simulink model "sampleModel2432"  (R2017a)
settings: Solver=VariableStepAuto  StartTime=0.0  StopTime=10.0  RelTol=1e-3
undefined symbols (not defined in the file or in its folder): DiscIntNeverNeededParam, sigbuilder_block
libraries: simulink x354
(part 1 of 6)
settings Model: Creator=cyfuzz  LastModifiedBy=cyfuzz

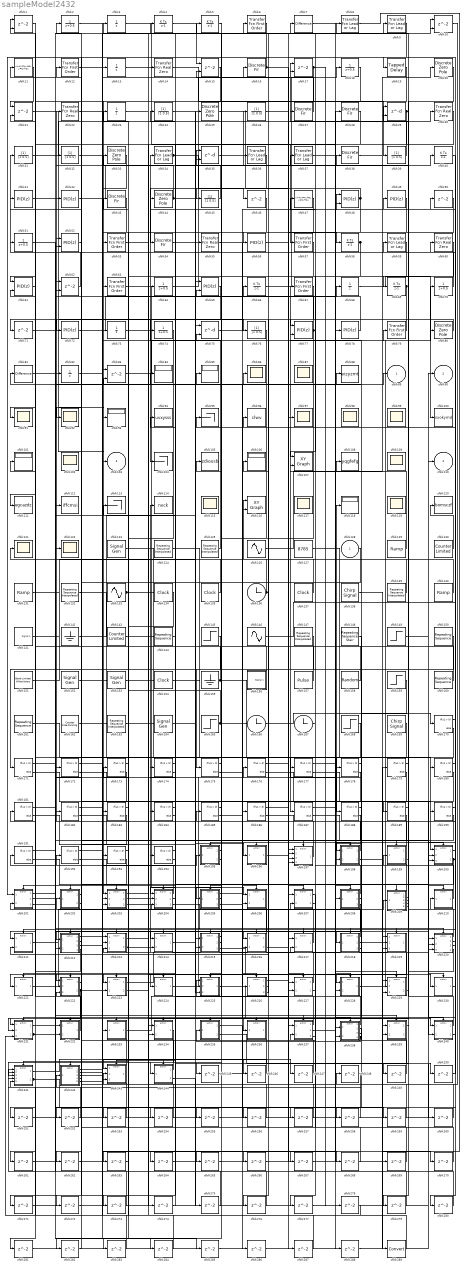
== system sampleModel2432 ==
  cfblk128 : Inport
  cfblk{1,10,15,17,21,62,83} (7 alike) : Delay  ShowEnablePort=on  SampleTime=1
      settings: InputPortMap=u0,e6
  cfblk100 : ToWorkspace  VariableName=sxokymd  SaveFormat=Timeseries  SampleTime=-1
  cfblk{84..85,93,101,106,118} (6 alike) : Display
  cfblk{86..87,91..92,97..99,102,109,115,117,119,121..122} (14 alike) : Scope
      cfblk102 settings: Floating=on
      cfblk109 settings: Floating=on
      cfblk115 settings: Floating=on
      cfblk117 settings: Floating=on
      cfblk119 settings: Floating=on
      cfblk87 settings: Floating=on
      cfblk98 settings: Floating=on
      cfblk99 settings: Floating=on
  cfblk104 : Terminator
  cfblk105 : ToWorkspace  VariableName=zdioxsb  SaveFormat=Timeseries  SampleTime=-1
  cfblk107 : simulink/Sinks/XY Graph  xmin=-1  xmax=1  ymin=-1  ymax=1  st=-1
  cfblk108 : ToWorkspace  VariableName=yqgfefg  SaveFormat=Timeseries  SampleTime=-1
  cfblk11 : DiscreteStateSpace
  cfblk111 : ToWorkspace  VariableName=egcazdz  SaveFormat=Timeseries  SampleTime=-1
  cfblk112 : ToWorkspace  VariableName=iffcmsi  SaveFormat=Timeseries  SampleTime=-1
  cfblk113 : Terminator
  cfblk114 : ToFile  Filename=nxck  SaveFormat=Timeseries
  cfblk116 : simulink/Sinks/XY Graph  xmin=-1  xmax=1  ymin=-1  ymax=1  st=-1
  cfblk{6,12,53,57,63,67,79} (7 alike) : simulink/Discrete/Transfer Fcn First Order  PoleZ=0.95  ICPrevOutput=0.0  DoSatur=off
      settings: SourceProductName=Simulink
  cfblk120 : ToWorkspace  VariableName=bomsczf  SaveFormat=Timeseries  SampleTime=-1
  cfblk{123,152..153,164} (4 alike) : SignalGenerator  Units=rad/sec
  cfblk{124..125,132,139,147,163} (6 alike) : simulink/Sources/Repeating Sequence Interpolated  OutValues=[3 1 4 2 1].'  TimeValues=[0 0.1 0.5 0.6 1].'  LookUpMeth=Interpolation-Use End Values  tsamp=0.01  OutMin=[]  OutMax=[]  OutDataTypeStr=double  OutputDataTypeScalingMode=double  OutDataType=fixdt(0,8)  OutScaling=2^-10
  cfblk126 : Sin  SampleTime=0
  cfblk127 : Constant  Value=8785
  cfblk129 : simulink/Sources/Ramp  slope=1  start=0  X0=0
  cfblk{3,13,23,68,73,82} (6 alike) : UnitDelay
  cfblk130 : simulink/Sources/Counter Limited  uplimit=7  tsamp=-1
  cfblk131 : simulink/Sources/Ramp  slope=1  start=0  X0=0
  cfblk133 : Sin  SampleTime=0
  cfblk{134..135,137,154} (4 alike) : DigitalClock
  cfblk136 : Clock
  cfblk138 : simulink/Sources/Chirp Signal  f1=0.1  T=100  f2=1
  cfblk{14,22,30,55,60} (5 alike) : simulink/Discrete/Transfer Fcn Real Zero  ZeroZ=0.75  ICPrevInput=0.0  DoSatur=off
      settings: SourceProductName=Simulink  SourceProductBaseCode=SL
  cfblk140 : simulink/Sources/Ramp  slope=1  start=0  X0=0
  cfblk141 : Subsystem  Tag=STV Subsys  LoadFcn=sigbuilder_block('load');  StartFcn=sigbuilder_block('start');  StopFcn=sigbuilder_block('stop');  ClipboardFcn=sigbuilder_block('clipboard');  mask(Sigbuilder block){tuvar=[0:10]}
      mask help: Simulink:masks:SigbuilderBlock_MD
      mask init:
      | if ~strcmp(get_param(bdroot(gcbh),'SimulationStatus'),'stopped') tuvar = sigbuilder_block('maskInit'); end
      settings: CopyFcn=sigbuilder_block('copy');  DeleteFcn=sigbuilder_block('delete');  ModelCloseFcn=sigbuilder_block('modelClose');  PreSaveFcn=sigbuilder_block('preSave');  PauseFcn=sigbuilder_block('pause');  ContinueFcn=sigbuilder_block('continue');  NameChangeFcn=sigbuilder_block('namechange');  OpenFcn=sigbuilder_block('open',[437.6 199.2 550.4 400 ]);  CloseFcn=sigbuilder_block('close');
      mask Display: plot(0, 0, 100, 100,[2, 2, 32, 32, 2], [68, 8, 8, 68, 68],[32, 2], [38, 38], [32, 19, 2],[53, 60, 44], [32, 17, 17, 2],[16, 16, 31, 31]);txt = getActiveGroup(gcbh);text(2, 100, txt,'verticalAlignment', 'top');
  cfblk142 : Ground
  cfblk143 : simulink/Sources/Counter Limited  uplimit=7  tsamp=-1
  cfblk{144,150,160..161} (4 alike) : simulink/Sources/Repeating Sequence  rep_seq_t=[0 2]  rep_seq_y=[0 2]
  cfblk145 : Step  After=94  SampleTime=0
  cfblk146 : Sin  SampleTime=0
  cfblk148 : simulink/Sources/Repeating Sequence Stair  OutValues=[3 1 4 2 1].'  tsamp=-1  OutMin=[]  OutMax=[]  OutDataTypeStr=double  OutputDataTypeScalingMode=double  OutDataType=fixdt(0,8)  ConRadixGroup=Best Precision: Vector-wise  OutScaling=2^-12
  cfblk149 : Step  After=59  SampleTime=0
  cfblk151 : simulink/Sources/Band-Limited White Noise  Cov=[0.1]  Ts=0.1  seed=[23341]
  cfblk155 : Ground
  cfblk156 : Subsystem  Tag=STV Subsys  LoadFcn=sigbuilder_block('load');  StartFcn=sigbuilder_block('start');  StopFcn=sigbuilder_block('stop');  ClipboardFcn=sigbuilder_block('clipboard');  mask(Sigbuilder block){tuvar=[0:10]}
      mask help: Simulink:masks:SigbuilderBlock_MD
      mask init:
      | if ~strcmp(get_param(bdroot(gcbh),'SimulationStatus'),'stopped') tuvar = sigbuilder_block('maskInit'); end
      settings: CopyFcn=sigbuilder_block('copy');  DeleteFcn=sigbuilder_block('delete');  ModelCloseFcn=sigbuilder_block('modelClose');  PreSaveFcn=sigbuilder_block('preSave');  PauseFcn=sigbuilder_block('pause');  ContinueFcn=sigbuilder_block('continue');  NameChangeFcn=sigbuilder_block('namechange');  OpenFcn=sigbuilder_block('open',[437.6 199.2 550.4 400 ]);  CloseFcn=sigbuilder_block('close');
      mask Display: plot(0, 0, 100, 100,[2, 2, 32, 32, 2], [68, 8, 8, 68, 68],[32, 2], [38, 38], [32, 19, 2],[53, 60, 44], [32, 17, 17, 2],[16, 16, 31, 31]);txt = getActiveGroup(gcbh);text(2, 100, txt,'verticalAlignment', 'top');
  cfblk157 : DiscretePulseGenerator  PulseType=Time based  Period=10  PulseWidth=5
  cfblk158 : UniformRandomNumber  SampleTime=0.1
  cfblk159 : Step  After=53  SampleTime=0
  cfblk{16,27..28,38,43,54} (6 alike) : DiscreteFir  SampleTime=1
  cfblk162 : simulink/Sources/Counter Free-Running  NumBits=16  tsamp=-1
  cfblk165 : Step  After=66  SampleTime=0
  cfblk166 : Clock
  cfblk167 : Clock
  cfblk168 : Step  After=29  SampleTime=0
  cfblk169 : simulink/Sources/Chirp Signal  f1=0.1  T=100  f2=1
  cfblk{170..194} (25 alike) : If  SampleTime=1
  cfblk{2,18,51,64,70,74} (6 alike) : DiscreteTransferFcn  SampleTime=1
  cfblk19 : simulink/Discrete/Tapped Delay  vinit=0.0  samptime=-1  NumDelays=1  DelayOrder=Oldest  includeCurrent=off
  cfblk195 : Subsystem  TreatAsAtomicUnit=on
  cfblk196 : Subsystem  TreatAsAtomicUnit=on
  cfblk197 : Subsystem  TreatAsAtomicUnit=on
  cfblk198 : Subsystem  TreatAsAtomicUnit=on
  cfblk199 : Subsystem  TreatAsAtomicUnit=on
  cfblk{20,25,33,44,80} (5 alike) : DiscreteZeroPole  Poles=[0 0.5]  Gain=1
  cfblk200 : Subsystem  TreatAsAtomicUnit=on
  cfblk201 : Subsystem  TreatAsAtomicUnit=on
  cfblk202 : Subsystem  TreatAsAtomicUnit=on
  cfblk203 : Subsystem  TreatAsAtomicUnit=on
  cfblk204 : Subsystem  TreatAsAtomicUnit=on
  cfblk205 : Subsystem  TreatAsAtomicUnit=on
  cfblk206 : Subsystem  TreatAsAtomicUnit=on
  cfblk207 : Subsystem  TreatAsAtomicUnit=on
  cfblk208 : Subsystem  TreatAsAtomicUnit=on
  cfblk209 : Subsystem  TreatAsAtomicUnit=on
  cfblk210 : Subsystem  TreatAsAtomicUnit=on
  cfblk211 : Subsystem  TreatAsAtomicUnit=on
  cfblk212 : Subsystem  TreatAsAtomicUnit=on
  cfblk213 : Subsystem  TreatAsAtomicUnit=on
  cfblk214 : Subsystem  TreatAsAtomicUnit=on
  cfblk215 : Subsystem  TreatAsAtomicUnit=on
  cfblk216 : Subsystem  TreatAsAtomicUnit=on
  cfblk217 : Subsystem  TreatAsAtomicUnit=on
  cfblk218 : Subsystem  TreatAsAtomicUnit=on
  cfblk219 : Subsystem  TreatAsAtomicUnit=on
  cfblk220 : Subsystem  TreatAsAtomicUnit=on
  cfblk221 : Subsystem  TreatAsAtomicUnit=on
  cfblk222 : Subsystem  TreatAsAtomicUnit=on
  cfblk223 : Subsystem  TreatAsAtomicUnit=on
  cfblk224 : Subsystem  TreatAsAtomicUnit=on
  cfblk225 : Subsystem  TreatAsAtomicUnit=on
  cfblk226 : Subsystem  TreatAsAtomicUnit=on
  cfblk227 : Subsystem  TreatAsAtomicUnit=on
  cfblk228 : Subsystem  TreatAsAtomicUnit=on
  cfblk229 : Subsystem  TreatAsAtomicUnit=on
  cfblk230 : Subsystem  TreatAsAtomicUnit=on
  cfblk231 : Subsystem  TreatAsAtomicUnit=on
  cfblk232 : Subsystem  TreatAsAtomicUnit=on
  cfblk233 : Subsystem  TreatAsAtomicUnit=on
  cfblk234 : Subsystem  TreatAsAtomicUnit=on
  cfblk235 : Subsystem  TreatAsAtomicUnit=on
  cfblk236 : Subsystem  TreatAsAtomicUnit=on
  cfblk237 : Subsystem  TreatAsAtomicUnit=on
  cfblk238 : Subsystem  TreatAsAtomicUnit=on
  cfblk239 : Subsystem  TreatAsAtomicUnit=on
  cfblk{24,26,31..32,39,45,76} (7 alike) : DiscreteFilter  SampleTime=1
  cfblk240 : Subsystem  TreatAsAtomicUnit=on
  cfblk241 : Subsystem  TreatAsAtomicUnit=on
  cfblk242 : Subsystem  TreatAsAtomicUnit=on
  cfblk243 : Subsystem  TreatAsAtomicUnit=on
  cfblk244 : Subsystem  TreatAsAtomicUnit=on
  cfblk{46,50,71,245..288} (47 alike) : Delay  SampleTime=1
  cfblk289 : DataTypeConversion
  cfblk29 : Delay  DelayLengthSource=Input port  SampleTime=1
      settings: InputPortMap=u0,p1
  cfblk{8..9,34,36..37,59} (6 alike) : simulink/Discrete/Transfer Fcn Lead or Lag  PoleZ=0.95  ZeroZ=0.75  ICPrevOutput=0.0  ICPrevInput=0.0  DoSatur=off
      settings: SourceProductName=Simulink  SourceProductBaseCode=SL
  cfblk35 : Delay  DelayLengthSource=Input port  SampleTime=1
      settings: InputPortMap=u0,p1
  cfblk{4..5,40,58,66,69} (6 alike) : DiscreteIntegrator  InitialConditionSetting=State (most efficient)  ICPrevOutput=DiscIntNeverNeededParam  ICPrevScaledInput=DiscIntNeverNeededParam
  cfblk{41..42,49,56,72,78} (6 alike) : simulink/Continuous/PID Controller  Controller=PID  TimeDomain=Discrete-time  SampleTime=1  IntegratorMethod=Forward Euler  FilterMethod=Forward Euler  Form=Parallel  UseFilter=on  ControllerParametersSource=internal  P=1  I=1  D=0  N=100  InitialConditionSource=internal  InitialConditionForIntegrator=0  InitialConditionForFilter=0  ExternalReset=none  LimitOutput=off  UpperSaturationLimit=inf  LowerSaturationLimit=-inf  LinearizeAsGain=off  AntiWindupMode=none  Kb=1  TrackingMode=off  Kt=1  PParamMin=[]  PParamMax=[]  IParamMin=[]  IParamMax=[]  DParamMin=[]  DParamMax=[]  NParamMin=[]  NParamMax=[]  KbParamMin=[]  KbParamMax=[]  KtParamMin=[]  KtParamMax=[]  POutMin=[]  POutMax=[]  IOutMin=[]  IOutMax=[]  DOutMin=[]  DOutMax=[]  NOutMin=[]  NOutMax=[]  KbOutMin=[]  KbOutMax=[]  KtOutMin=[]  KtOutMax=[]  IntegratorOutMin=[]  IntegratorOutMax=[]  FilterOutMin=[]  FilterOutMax=[]  SumOutMin=[]  SumOutMax=[]  SumI1OutMin=[]  SumI1OutMax=[]  SumI2OutMin=[]  SumI2OutMax=[]  SumI3OutMin=[]  SumI3OutMax=[]  SumDOutMin=[]  SumDOutMax=[]  SaturationOutMin=[]  SaturationOutMax=[]  IntegratorContinuousStateAttributes=''  IntegratorStateMustResolveToSignalObject=off  IntegratorRTWStateStorageClass=Auto  FilterContinuousStateAttributes=''  FilterStateMustResolveToSignalObject=off  FilterRTWStateStorageClass=Auto  DifferentiatorICPrevScaledInput=0  DifferentiatorOutMin=[]  DifferentiatorOutMax=[]  InitialConditionSetting=State (most efficient)
  cfblk47 : DiscreteStateSpace
  cfblk{48,52,61,65,77} (5 alike) : simulink/Continuous/PID Controller (2DOF)  Controller=PID  TimeDomain=Discrete-time  SampleTime=1  IntegratorMethod=Forward Euler  FilterMethod=Forward Euler  Form=Parallel  UseFilter=on  ControllerParametersSource=internal  P=1  I=1  D=0  N=100  b=1  c=1  InitialConditionSource=internal  InitialConditionForIntegrator=0  InitialConditionForFilter=0  ExternalReset=none  LimitOutput=off  UpperSaturationLimit=inf  LowerSaturationLimit=-inf  LinearizeAsGain=off  AntiWindupMode=none  Kb=1  TrackingMode=off  Kt=1  PParamMin=[]  PParamMax=[]  IParamMin=[]  IParamMax=[]  DParamMin=[]  DParamMax=[]  NParamMin=[]  NParamMax=[]  bParamMin=[]  bParamMax=[]  cParamMin=[]  cParamMax=[]  KbParamMin=[]  KbParamMax=[]  KtParamMin=[]  KtParamMax=[]  POutMin=[]  POutMax=[]  IOutMin=[]  IOutMax=[]  DOutMin=[]  DOutMax=[]  NOutMin=[]  NOutMax=[]  bOutMin=[]  bOutMax=[]  cOutMin=[]  cOutMax=[]  KbOutMin=[]  KbOutMax=[]  KtOutMin=[]  KtOutMax=[]  IntegratorOutMin=[]  IntegratorOutMax=[]  FilterOutMin=[]  FilterOutMax=[]  SumOutMin=[]  SumOutMax=[]  Sum1OutMin=[]  Sum1OutMax=[]  Sum2OutMin=[]  Sum2OutMax=[]  Sum3OutMin=[]  Sum3OutMax=[]  SumI1OutMin=[]  SumI1OutMax=[]  SumI2OutMin=[]  SumI2OutMax=[]  SumI3OutMin=[]  SumI3OutMax=[]  SumDOutMin=[]  SumDOutMax=[]  SaturationOutMin=[]  SaturationOutMax=[]  IntegratorContinuousStateAttributes=''  IntegratorStateMustResolveToSignalObject=off  IntegratorRTWStateStorageClass=Auto  FilterContinuousStateAttributes=''  FilterStateMustResolveToSignalObject=off  FilterRTWStateStorageClass=Auto  DifferentiatorICPrevScaledInput=0  DifferentiatorOutMin=[]  DifferentiatorOutMax=[]  InitialConditionSetting=State (most efficient)
  cfblk7 : simulink/Discrete/Difference  ICPrevInput=0.0  OutMin=[]  OutMax=[]  OutDataTypeStr=Inherit: Inherit via back propagation  OutDataType=fixdt(1, 16)  OutScaling=2^-10  DoSatur=off
  cfblk75 : Delay  DelayLengthSource=Input port  SampleTime=1
      settings: InputPortMap=u0,p1
  cfblk81 : simulink/Discrete/Difference  ICPrevInput=0.0  OutMin=[]  OutMax=[]  OutDataTypeStr=Inherit: Inherit via back propagation  OutDataType=fixdt(1, 16)  OutScaling=2^-10  DoSatur=off
  cfblk88 : ToWorkspace  VariableName=eizyzmt  SaveFormat=Timeseries  SampleTime=-1
  cfblk94 : ToWorkspace  VariableName=uvxysss  SaveFormat=Timeseries  SampleTime=-1
  cfblk95 : Terminator
  cfblk96 : ToFile  Filename=clwv  SaveFormat=Timeseries
  cfblk89 : Outport
  cfblk90 : Outport  Port=2
  cfblk103 : Outport  Port=3
  cfblk110 : Outport  Port=4
  wires:
  cfblk64/1 -> cfblk16/1
  cfblk66/1 -> cfblk18/1
  cfblk43/1 -> cfblk203/1(cfblk1)
  cfblk69/1 -> cfblk262/1, cfblk272/1
  cfblk68/1 -> cfblk100/1
  cfblk33/1 -> cfblk193/1
  cfblk137/1 -> cfblk116/1
  cfblk225/1(cfblk2) -> cfblk240/1(cfblk1)
  cfblk166/1 -> cfblk170/1
  cfblk21/1 -> cfblk76/1
  cfblk136/1 -> cfblk121/1, cfblk216/1(cfblk1)
  cfblk83/1 -> cfblk79/1
  cfblk19/1 -> cfblk83/1
  cfblk63/1 -> cfblk206/1(cfblk1)
  cfblk146/1 -> cfblk19/1
  cfblk150/1 -> cfblk175/1
  cfblk16/1 -> cfblk201/1(cfblk1), cfblk229/2(cfblk12)
  cfblk228/1(cfblk2) -> cfblk70/1
  cfblk4/1 -> cfblk15/1
  cfblk165/1 -> cfblk200/1(cfblk1), cfblk43/1, cfblk227/1(cfblk1)
  cfblk224/1(cfblk2) -> cfblk67/1
  cfblk230/1(cfblk2) -> cfblk50/1
  cfblk41/1 -> cfblk93/1
  cfblk202/1(cfblk2) -> cfblk181/1
  cfblk125/1 -> cfblk34/1
  cfblk5/1 -> cfblk205/1(cfblk1)
  cfblk199/1(cfblk2) -> cfblk85/1
  cfblk58/1 -> cfblk107/1, cfblk227/2(cfblk11)
  cfblk164/1 -> cfblk55/1
  cfblk62/1 -> cfblk31/1
  cfblk221/1(cfblk2) -> cfblk25/1
  cfblk210/1(cfblk2) -> cfblk199/1(cfblk1)
  cfblk207/1(cfblk2) -> cfblk224/1(cfblk1)
  cfblk149/1 -> cfblk90/1
  cfblk39/1 -> cfblk17/1
  cfblk227/1(cfblk2) -> cfblk113/1
  cfblk71/1 -> cfblk103/1
  cfblk73/1 -> cfblk104/1
  cfblk131/1 -> cfblk75/1
  cfblk198/1(cfblk2) -> cfblk22/1
  cfblk52/1 -> cfblk11/1
  cfblk151/1 -> cfblk13/1
  cfblk229/1(cfblk2) -> cfblk114/1
  cfblk82/1 -> cfblk17/2
  cfblk34/1 -> cfblk46/1, cfblk220/3(cfblk11)
  cfblk54/1 -> cfblk218/1(cfblk1)
  cfblk36/1 -> cfblk54/1
  cfblk209/1(cfblk2) -> cfblk27/1
  cfblk1/1 -> cfblk71/1
  cfblk75/1 -> cfblk48/1
  cfblk78/1 -> cfblk2/1
  cfblk234/1(cfblk2) -> cfblk243/2(cfblk11)
  cfblk14/1 -> cfblk39/1
  cfblk18/1 -> cfblk203/3(cfblk14)
  cfblk129/1 -> cfblk107/2
  cfblk3/1 -> cfblk57/1
  cfblk208/1(cfblk2) -> cfblk118/1
  cfblk205/1(cfblk2) -> cfblk240/2(cfblk7)
  cfblk206/1(cfblk2) -> cfblk214/1(cfblk1)
  cfblk133/1 -> cfblk226/1(cfblk1), cfblk197/4(cfblk16)
  cfblk218/1(cfblk2) -> cfblk52/1
  cfblk42/1 -> cfblk37/1
  cfblk156/1(Signal 1) -> cfblk82/1
  cfblk48/1 -> cfblk204/1(cfblk1), cfblk45/1
  cfblk2/1 -> cfblk63/1
  cfblk123/1 -> cfblk238/1(cfblk1)
  cfblk223/1(cfblk2) -> cfblk110/1
  cfblk11/1 -> cfblk21/1
  cfblk70/1 -> cfblk21/2
  cfblk219/1(cfblk2) -> cfblk221/1(cfblk1)
  cfblk29/1 -> cfblk61/1, cfblk69/1
  cfblk139/1 -> cfblk108/1
  cfblk199/2(cfblk11) -> cfblk59/1
  cfblk242/1(cfblk2) -> cfblk38/1
  cfblk59/1 -> cfblk77/1
  cfblk79/1 -> cfblk72/1
  cfblk212/1(cfblk2) -> cfblk40/1
  cfblk153/1 -> cfblk188/1
  cfblk24/1 -> cfblk196/1(cfblk1)
  cfblk37/1 -> cfblk190/1
  cfblk154/1 -> cfblk187/1
  cfblk128/1 -> cfblk222/1(cfblk1)
  cfblk132/1 -> cfblk180/1
  cfblk124/1 -> cfblk207/1(cfblk1)
  cfblk13/1 -> cfblk78/1
  cfblk141/1(Signal 1) -> cfblk64/1
  cfblk25/1 -> cfblk237/1(cfblk1)
  cfblk152/1 -> cfblk238/2(cfblk12)
  cfblk242/2(cfblk14) -> cfblk195/1(cfblk1)
  cfblk135/1 -> cfblk94/1
  cfblk77/1 -> cfblk7/1, cfblk35/2, cfblk255/1
  cfblk46/1 -> cfblk53/1
  cfblk240/1(cfblk2) -> cfblk29/1
  cfblk195/2(cfblk7) -> cfblk44/1
  cfblk26/1 -> cfblk58/1
  cfblk127/1 -> cfblk219/1(cfblk1)
  cfblk72/1 -> cfblk66/1
  cfblk148/1 -> cfblk198/1(cfblk1)
  cfblk27/1 -> cfblk15/2
  cfblk38/1 -> cfblk20/1
  cfblk81/1 -> cfblk236/1(cfblk1)
  cfblk9/1 -> cfblk92/1
  cfblk50/1 -> cfblk56/1
  cfblk126/1 -> cfblk29/2
  cfblk203/2(cfblk15) -> cfblk68/1
  cfblk213/2(cfblk9) -> cfblk201/2(cfblk11), cfblk225/3(cfblk15)
  cfblk32/1 -> cfblk73/1
  cfblk203/3(cfblk16) -> cfblk207/2(cfblk8)
  cfblk204/1(cfblk2) -> cfblk101/1
  cfblk31/1 -> cfblk30/1
  cfblk80/1 -> cfblk74/1
  cfblk202/2(cfblk9) -> cfblk122/1
  cfblk138/1 -> cfblk239/1(cfblk1)
  cfblk233/1(cfblk2) -> cfblk197/1(cfblk1)
  cfblk238/1(cfblk2) -> cfblk4/1
  cfblk161/1 -> cfblk208/1(cfblk1)
  cfblk229/2(cfblk14) -> cfblk6/1
  cfblk12/1 -> cfblk9/1
  cfblk145/1 -> cfblk171/1
  cfblk157/1 -> cfblk106/1
  cfblk211/1(cfblk2) -> cfblk186/1
  cfblk57/1 -> cfblk116/2
  cfblk35/1 -> cfblk26/1
  cfblk17/1 -> cfblk91/1, cfblk278/1
  cfblk45/1 -> cfblk24/1
  cfblk158/1 -> cfblk1/1
  cfblk240/2(cfblk8) -> cfblk49/1
  cfblk241/2(cfblk12) -> cfblk84/1, cfblk286/1
  cfblk242/3(cfblk15) -> cfblk80/1
  cfblk47/1 -> cfblk197/2(cfblk14)
  cfblk208/2(cfblk7) -> cfblk77/2
  cfblk212/2(cfblk10) -> cfblk32/1
  cfblk243/1(cfblk2) -> cfblk182/1
  cfblk140/1 -> cfblk61/2
  cfblk15/1 -> cfblk111/1
  cfblk214/1(cfblk2) -> cfblk209/1(cfblk1)
  cfblk197/1(cfblk2) -> cfblk23/1
  cfblk134/1 -> cfblk223/1(cfblk1)
  cfblk53/1 -> cfblk36/1
  cfblk220/1(cfblk2) -> cfblk96/1
  cfblk223/2(cfblk9) -> cfblk14/1
  cfblk220/2(cfblk12) -> cfblk184/1
  cfblk205/2(cfblk7) -> cfblk105/1
  cfblk160/1 -> cfblk5/1
  cfblk167/1 -> cfblk47/1
  cfblk205/3(cfblk8) -> cfblk89/1
  cfblk144/1 -> cfblk244/1(cfblk1)
  cfblk23/1 -> cfblk8/1
  cfblk168/1 -> cfblk211/1(cfblk1)
  cfblk244/1(cfblk2) -> cfblk42/1
  cfblk44/1 -> cfblk12/1, cfblk228/2(cfblk8)
  cfblk142/1 -> cfblk65/1
  cfblk204/2(cfblk11) -> cfblk112/1
  cfblk216/1(cfblk2) -> cfblk51/1
  cfblk232/1(cfblk2) -> cfblk1/2
  cfblk155/1 -> cfblk83/2, cfblk229/3(cfblk13)
  cfblk215/1(cfblk2) -> cfblk241/3(cfblk9)
  cfblk227/2(cfblk12) -> cfblk65/2
  cfblk163/1 -> cfblk197/3(cfblk15)
  cfblk212/3(cfblk11) -> cfblk223/2(cfblk8)
  cfblk200/2(cfblk10) -> cfblk60/1, cfblk254/1
  cfblk231/1(cfblk2) -> cfblk10/1
  cfblk215/2(cfblk11) -> cfblk185/1
  cfblk217/1(cfblk2) -> cfblk62/1
  cfblk143/1 -> cfblk229/1(cfblk1)
  cfblk169/1 -> cfblk214/2(cfblk9)
  cfblk196/1(cfblk2) -> cfblk10/2
  cfblk216/2(cfblk14) -> cfblk178/1
  cfblk222/1(cfblk2) -> cfblk232/2(cfblk7)
  cfblk55/1 -> cfblk189/1
  cfblk242/4(cfblk16) -> cfblk41/1
  cfblk226/1(cfblk2) -> cfblk97/1
  cfblk28/1 -> cfblk204/3(cfblk10)
  cfblk6/1 -> cfblk231/1(cfblk1)
  cfblk208/3(cfblk8) -> cfblk212/1(cfblk1)
  cfblk226/2(cfblk14) -> cfblk211/2(cfblk7)
  cfblk201/1(cfblk2) -> cfblk215/2(cfblk10)
  cfblk209/3(cfblk5) -> cfblk234/2(cfblk7)
  cfblk238/4(cfblk15) -> cfblk235/1(cfblk1), cfblk225/1(cfblk1)
  cfblk159/1 -> cfblk228/1(cfblk1)
  cfblk226/3(cfblk15) -> cfblk3/1
  cfblk209/4(cfblk6) -> cfblk35/1
  cfblk215/3(cfblk12) -> cfblk230/1(cfblk1)
  cfblk209/5(cfblk7) -> cfblk48/2
  cfblk237/1(cfblk2) -> cfblk75/2
  cfblk231/2(cfblk13) -> cfblk176/1, cfblk285/1
  cfblk147/1 -> cfblk212/2(cfblk9)
  cfblk201/2(cfblk12) -> cfblk62/2
  cfblk201/3(cfblk13) -> cfblk88/1
  cfblk237/2(cfblk14) -> cfblk28/1
  cfblk130/1 -> cfblk120/1
  cfblk237/3(cfblk15) -> cfblk52/2
  cfblk222/2(cfblk8) -> cfblk231/2(cfblk11), cfblk86/1
  cfblk220/3(cfblk13) -> cfblk95/1
  cfblk218/3(cfblk17) -> cfblk81/1
  cfblk170/1 -> cfblk195/Action
  cfblk170/2 -> cfblk196/Action
  cfblk171/1 -> cfblk197/Action
  cfblk171/2 -> cfblk198/Action
  cfblk172/1 -> cfblk199/Action
  cfblk172/2 -> cfblk200/Action
  cfblk173/1 -> cfblk201/Action
  cfblk173/2 -> cfblk202/Action
  cfblk174/1 -> cfblk203/Action
  cfblk174/2 -> cfblk204/Action
  cfblk175/1 -> cfblk205/Action
  cfblk175/2 -> cfblk206/Action
  cfblk176/1 -> cfblk207/Action
  cfblk176/2 -> cfblk208/Action
  cfblk177/1 -> cfblk209/Action
  cfblk177/2 -> cfblk210/Action
  cfblk178/1 -> cfblk211/Action
  cfblk178/2 -> cfblk212/Action
  cfblk179/1 -> cfblk213/Action
  cfblk179/2 -> cfblk214/Action
  cfblk180/1 -> cfblk215/Action
  cfblk180/2 -> cfblk216/Action
  cfblk181/1 -> cfblk217/Action
  cfblk181/2 -> cfblk218/Action
  cfblk182/1 -> cfblk219/Action
  cfblk182/2 -> cfblk220/Action
  cfblk183/1 -> cfblk221/Action
  cfblk183/2 -> cfblk222/Action
  cfblk184/1 -> cfblk223/Action
  cfblk184/2 -> cfblk224/Action
  cfblk185/1 -> cfblk225/Action
  cfblk185/2 -> cfblk226/Action
  cfblk186/1 -> cfblk227/Action
  cfblk186/2 -> cfblk228/Action
  cfblk187/1 -> cfblk229/Action
  cfblk187/2 -> cfblk230/Action
  cfblk188/1 -> cfblk231/Action
  cfblk188/2 -> cfblk232/Action
  cfblk189/1 -> cfblk233/Action
  cfblk189/2 -> cfblk234/Action
  cfblk190/1 -> cfblk235/Action
  cfblk190/2 -> cfblk236/Action
  cfblk191/1 -> cfblk237/Action
  cfblk191/2 -> cfblk238/Action
  cfblk192/1 -> cfblk239/Action
  cfblk192/2 -> cfblk240/Action
  cfblk193/1 -> cfblk241/Action
  cfblk193/2 -> cfblk242/Action
  cfblk194/1 -> cfblk243/Action
  cfblk194/2 -> cfblk244/Action
  cfblk209/2(cfblk4) -> cfblk245/1
  cfblk245/1 -> cfblk206/2(cfblk10)
  cfblk213/1(cfblk2) -> cfblk246/1
  cfblk246/1 -> cfblk243/1(cfblk1)
  cfblk241/1(cfblk2) -> cfblk247/1
  cfblk247/1 -> cfblk222/3(cfblk7)
  cfblk10/1 -> cfblk248/1
  cfblk248/1 -> cfblk242/1(cfblk1)
  cfblk20/1 -> cfblk249/1
  cfblk249/1 -> cfblk177/1
  cfblk7/1 -> cfblk250/1
  cfblk250/1 -> cfblk210/1(cfblk1)
  cfblk65/1 -> cfblk251/1
  cfblk251/1 -> cfblk200/2(cfblk8)
  cfblk200/1(cfblk2) -> cfblk252/1
  cfblk252/1 -> cfblk241/1(cfblk1)
  cfblk60/1 -> cfblk253/1
  cfblk253/1 -> cfblk243/3(cfblk12)
  cfblk254/1 -> cfblk213/3(cfblk8)
  cfblk255/1 -> cfblk216/2(cfblk13)
  cfblk51/1 -> cfblk256/1
  cfblk256/1 -> cfblk191/1
  cfblk238/2(cfblk13) -> cfblk257/1
  cfblk257/1 -> cfblk234/1(cfblk1)
  cfblk238/3(cfblk14) -> cfblk258/1
  cfblk258/1 -> cfblk241/4(cfblk10)
  cfblk235/1(cfblk2) -> cfblk259/1
  cfblk259/1 -> cfblk237/2(cfblk13)
  cfblk235/2(cfblk8) -> cfblk260/1
  cfblk260/1 -> cfblk222/2(cfblk6)
  cfblk61/1 -> cfblk261/1
  cfblk261/1 -> cfblk183/1
  cfblk262/1 -> cfblk233/1(cfblk1)
  cfblk8/1 -> cfblk263/1
  cfblk263/1 -> cfblk173/1
  cfblk30/1 -> cfblk264/1
  cfblk264/1 -> cfblk215/1(cfblk1)
  cfblk76/1 -> cfblk265/1
  cfblk265/1 -> cfblk239/2(cfblk10)
  cfblk239/1(cfblk2) -> cfblk266/1
  cfblk266/1 -> cfblk217/1(cfblk1)
  cfblk239/2(cfblk11) -> cfblk267/1
  cfblk267/1 -> cfblk198/2(cfblk11)
  cfblk22/1 -> cfblk268/1
  cfblk268/1 -> cfblk217/2(cfblk7)
  cfblk198/2(cfblk12) -> cfblk269/1
  cfblk269/1 -> cfblk172/1
  cfblk218/2(cfblk16) -> cfblk270/1
  cfblk270/1 -> cfblk213/2(cfblk7)
  cfblk236/1(cfblk2) -> cfblk271/1
  cfblk271/1 -> cfblk200/3(cfblk9)
  cfblk272/1 -> cfblk225/2(cfblk14)
  cfblk49/1 -> cfblk273/1
  cfblk273/1 -> cfblk203/2(cfblk13)
  cfblk203/1(cfblk2) -> cfblk274/1
  cfblk274/1 -> cfblk194/1
  cfblk244/2(cfblk7) -> cfblk275/1
  cfblk275/1 -> cfblk192/1
  cfblk67/1 -> cfblk276/1
  cfblk276/1 -> cfblk241/2(cfblk8)
  cfblk207/2(cfblk9) -> cfblk277/1
  cfblk277/1 -> cfblk220/1(cfblk1)
  cfblk278/1 -> cfblk231/3(cfblk12)
  cfblk220/4(cfblk14) -> cfblk279/1
  cfblk279/1 -> cfblk174/1
  cfblk40/1 -> cfblk280/1
  cfblk280/1 -> cfblk232/1(cfblk1)
  cfblk212/4(cfblk12) -> cfblk281/1
  cfblk281/1 -> cfblk220/2(cfblk10)
  cfblk195/1(cfblk2) -> cfblk282/1
  cfblk282/1 -> cfblk202/1(cfblk1)
  cfblk74/1 -> cfblk283/1
  cfblk283/1 -> cfblk213/1(cfblk1)
  cfblk242/5(cfblk17) -> cfblk284/1
  cfblk284/1 -> cfblk241/5(cfblk11)
  cfblk285/1 -> cfblk219/3(cfblk9)
  cfblk286/1 -> cfblk219/2(cfblk8)
  cfblk56/1 -> cfblk287/1
  cfblk287/1 -> cfblk204/2(cfblk9)
  cfblk204/3(cfblk12) -> cfblk288/1
  cfblk288/1 -> cfblk179/1
  cfblk162/1 -> cfblk289/1
  cfblk289/1 -> cfblk33/1

== system sampleModel2432/cfblk141 ==
  Demux : Demux  Tag=STV Demux  Outputs=1
  FromWs : FromWorkspace  Tag=STV FromWs  VariableName=tuvar  SampleTime=0
      SigBuilderData=|
      | common.afterFinalStr = 'Extrapolate'
      | common.sampleTime = 0
      | dataSet.timeRange = [0 10]
      | dataSet.name = 'Group 1'
      | sbobj.Groups.Name = 'Group 1'
      | sbobj.Groups.Signals.Name = 'Signal 1'
      | sbobj.Groups.Signals.XData = [0 4 4 6 6 10]
      | sbobj.Groups.Signals.YData = [0 0 1 1 0 0]
  Signal 1 : Outport  Tag=STV Outport
  wires:
  Demux/1 -> Signal 1/1
  FromWs/1 -> Demux/1

== system sampleModel2432/cfblk156 ==
  Demux : Demux  Tag=STV Demux  Outputs=1
  FromWs : FromWorkspace  Tag=STV FromWs  VariableName=tuvar  SampleTime=0
      SigBuilderData=|
      | common.afterFinalStr = 'Extrapolate'
      | common.sampleTime = 0
      | dataSet.timeRange = [0 10]
      | dataSet.name = 'Group 1'
      | sbobj.Groups.Name = 'Group 1'
      | sbobj.Groups.Signals.Name = 'Signal 1'
      | sbobj.Groups.Signals.XData = [0 4 4 6 6 10]
      | sbobj.Groups.Signals.YData = [0 0 1 1 0 0]
  Signal 1 : Outport  Tag=STV Outport
  wires:
  Demux/1 -> Signal 1/1
  FromWs/1 -> Demux/1

== system sampleModel2432/cfblk195 ==
  cfblk1 : Inport
  Action Port : ActionPort  ActionType=then
  cfblk3 : Delay  DelayLengthSource=Input port
      settings: InputPortMap=u0,p1
  cfblk4 : DiscreteStateSpace  SampleTime=-1
  cfblk5 : DiscreteFilter
  cfblk6 : simulink/Continuous/PID Controller (2DOF)  Controller=PID  TimeDomain=Discrete-time  SampleTime=-1  IntegratorMethod=Forward Euler  FilterMethod=Forward Euler  Form=Parallel  UseFilter=on  ControllerParametersSource=internal  P=1  I=1  D=0  N=100  b=1  c=1  InitialConditionSource=internal  InitialConditionForIntegrator=0  InitialConditionForFilter=0  ExternalReset=none  LimitOutput=off  UpperSaturationLimit=inf  LowerSaturationLimit=-inf  LinearizeAsGain=off  AntiWindupMode=none  Kb=1  TrackingMode=off  Kt=1  PParamMin=[]  PParamMax=[]  IParamMin=[]  IParamMax=[]  DParamMin=[]  DParamMax=[]  NParamMin=[]  NParamMax=[]  bParamMin=[]  bParamMax=[]  cParamMin=[]  cParamMax=[]  KbParamMin=[]  KbParamMax=[]  KtParamMin=[]  KtParamMax=[]  POutMin=[]  POutMax=[]  IOutMin=[]  IOutMax=[]  DOutMin=[]  DOutMax=[]  NOutMin=[]  NOutMax=[]  bOutMin=[]  bOutMax=[]  cOutMin=[]  cOutMax=[]  KbOutMin=[]  KbOutMax=[]  KtOutMin=[]  KtOutMax=[]  IntegratorOutMin=[]  IntegratorOutMax=[]  FilterOutMin=[]  FilterOutMax=[]  SumOutMin=[]  SumOutMax=[]  Sum1OutMin=[]  Sum1OutMax=[]  Sum2OutMin=[]  Sum2OutMax=[]  Sum3OutMin=[]  Sum3OutMax=[]  SumI1OutMin=[]  SumI1OutMax=[]  SumI2OutMin=[]  SumI2OutMax=[]  SumI3OutMin=[]  SumI3OutMax=[]  SumDOutMin=[]  SumDOutMax=[]  SaturationOutMin=[]  SaturationOutMax=[]  IntegratorContinuousStateAttributes=''  IntegratorStateMustResolveToSignalObject=off  IntegratorRTWStateStorageClass=Auto  FilterContinuousStateAttributes=''  FilterStateMustResolveToSignalObject=off  FilterRTWStateStorageClass=Auto  DifferentiatorICPrevScaledInput=0  DifferentiatorOutMin=[]  DifferentiatorOutMax=[]  InitialConditionSetting=State (most efficient)
  cfblk8 : Delay
  cfblk2 : Outport
  cfblk7 : Outport  Port=2
  wires:
  cfblk3/1 -> cfblk2/1, cfblk5/1
  cfblk1/1 -> cfblk6/1, cfblk6/2
  cfblk5/1 -> cfblk4/1
  cfblk6/1 -> cfblk7/1, cfblk3/2
  cfblk4/1 -> cfblk8/1
  cfblk8/1 -> cfblk3/1

== system sampleModel2432/cfblk196 ==
  cfblk1 : Inport
  Action Port : ActionPort  ActionType=else
  cfblk{10,14..17} (5 alike) : Delay
  cfblk11 : If  SampleTime=1
  cfblk12 : Subsystem  TreatAsAtomicUnit=on
  cfblk13 : Subsystem  TreatAsAtomicUnit=on
  cfblk3 : DiscreteFir
  cfblk4 : DiscreteTransferFcn
  cfblk5 : simulink/Discrete/Tapped Delay  vinit=0.0  samptime=-1  NumDelays=1  DelayOrder=Oldest  includeCurrent=off
  cfblk6 : DiscreteFilter
  cfblk7 : DiscreteIntegrator  InitialConditionSetting=State (most efficient)  SampleTime=-1  ICPrevOutput=DiscIntNeverNeededParam  ICPrevScaledInput=DiscIntNeverNeededParam
  cfblk8 : simulink/Discrete/Transfer Fcn Real Zero  ZeroZ=0.75  ICPrevInput=0.0  DoSatur=off
      settings: SourceProductName=Simulink  SourceProductBaseCode=SL
  cfblk9 : Delay  DelayLengthSource=Input port
      settings: InputPortMap=u0,p1
  cfblk2 : Outport
  wires:
  cfblk6/1 -> cfblk9/1
  cfblk4/1 -> cfblk8/1
  cfblk8/1 -> cfblk10/1
  cfblk9/1 -> cfblk2/1
  cfblk1/1 -> cfblk12/1(cfblk1)
  cfblk13/1(cfblk2) -> cfblk3/1
  cfblk13/2(cfblk9) -> cfblk7/1
  cfblk12/1(cfblk2) -> cfblk4/1
  cfblk12/2(cfblk11) -> cfblk9/2
  cfblk12/3(cfblk12) -> cfblk6/1, cfblk5/1
  cfblk11/1 -> cfblk12/Action
  cfblk11/2 -> cfblk13/Action
  cfblk10/1 -> cfblk14/1
  cfblk14/1 -> cfblk11/1
  cfblk3/1 -> cfblk15/1
  cfblk15/1 -> cfblk13/2(cfblk8)
  cfblk7/1 -> cfblk16/1
  cfblk16/1 -> cfblk13/1(cfblk1)
  cfblk5/1 -> cfblk17/1
  cfblk17/1 -> cfblk12/2(cfblk10)

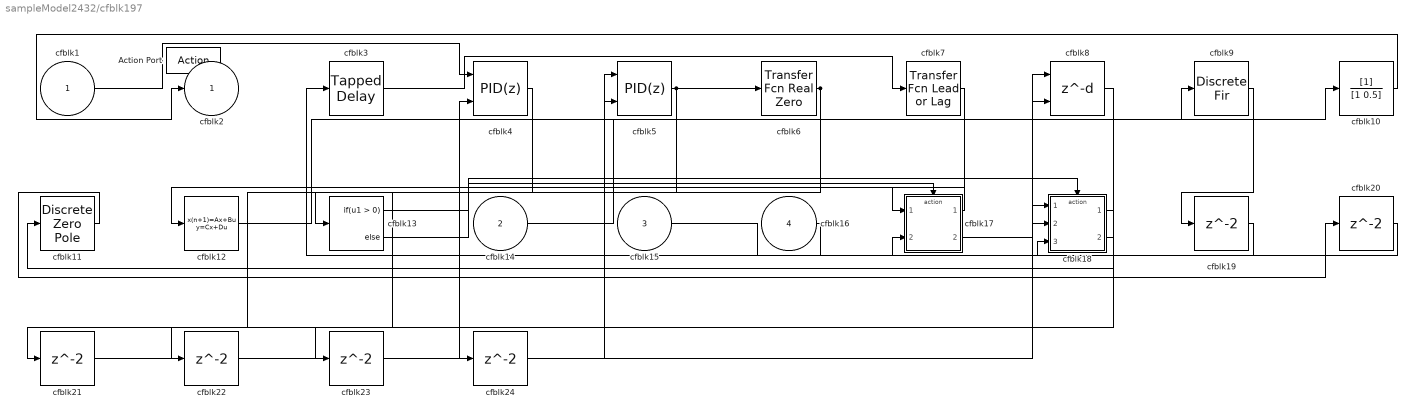
== system sampleModel2432/cfblk197 ==
  cfblk1 : Inport
  cfblk14 : Inport  Port=2
  cfblk15 : Inport  Port=3
  cfblk16 : Inport  Port=4
  Action Port : ActionPort  ActionType=then
  cfblk10 : DiscreteFilter
  cfblk11 : DiscreteZeroPole  Poles=[0 0.5]  Gain=1  SampleTime=-1
  cfblk12 : DiscreteStateSpace  SampleTime=-1
  cfblk13 : If  SampleTime=1
  cfblk17 : Subsystem  TreatAsAtomicUnit=on
  cfblk18 : Subsystem  TreatAsAtomicUnit=on
  cfblk{19..24} (6 alike) : Delay
  cfblk3 : simulink/Discrete/Tapped Delay  vinit=0.0  samptime=-1  NumDelays=1  DelayOrder=Oldest  includeCurrent=off
  cfblk4 : simulink/Continuous/PID Controller (2DOF)  Controller=PID  TimeDomain=Discrete-time  SampleTime=-1  IntegratorMethod=Forward Euler  FilterMethod=Forward Euler  Form=Parallel  UseFilter=on  ControllerParametersSource=internal  P=1  I=1  D=0  N=100  b=1  c=1  InitialConditionSource=internal  InitialConditionForIntegrator=0  InitialConditionForFilter=0  ExternalReset=none  LimitOutput=off  UpperSaturationLimit=inf  LowerSaturationLimit=-inf  LinearizeAsGain=off  AntiWindupMode=none  Kb=1  TrackingMode=off  Kt=1  PParamMin=[]  PParamMax=[]  IParamMin=[]  IParamMax=[]  DParamMin=[]  DParamMax=[]  NParamMin=[]  NParamMax=[]  bParamMin=[]  bParamMax=[]  cParamMin=[]  cParamMax=[]  KbParamMin=[]  KbParamMax=[]  KtParamMin=[]  KtParamMax=[]  POutMin=[]  POutMax=[]  IOutMin=[]  IOutMax=[]  DOutMin=[]  DOutMax=[]  NOutMin=[]  NOutMax=[]  bOutMin=[]  bOutMax=[]  cOutMin=[]  cOutMax=[]  KbOutMin=[]  KbOutMax=[]  KtOutMin=[]  KtOutMax=[]  IntegratorOutMin=[]  IntegratorOutMax=[]  FilterOutMin=[]  FilterOutMax=[]  SumOutMin=[]  SumOutMax=[]  Sum1OutMin=[]  Sum1OutMax=[]  Sum2OutMin=[]  Sum2OutMax=[]  Sum3OutMin=[]  Sum3OutMax=[]  SumI1OutMin=[]  SumI1OutMax=[]  SumI2OutMin=[]  SumI2OutMax=[]  SumI3OutMin=[]  SumI3OutMax=[]  SumDOutMin=[]  SumDOutMax=[]  SaturationOutMin=[]  SaturationOutMax=[]  IntegratorContinuousStateAttributes=''  IntegratorStateMustResolveToSignalObject=off  IntegratorRTWStateStorageClass=Auto  FilterContinuousStateAttributes=''  FilterStateMustResolveToSignalObject=off  FilterRTWStateStorageClass=Auto  DifferentiatorICPrevScaledInput=0  DifferentiatorOutMin=[]  DifferentiatorOutMax=[]  InitialConditionSetting=State (most efficient)
  cfblk5 : simulink/Continuous/PID Controller (2DOF)  Controller=PID  TimeDomain=Discrete-time  SampleTime=-1  IntegratorMethod=Forward Euler  FilterMethod=Forward Euler  Form=Parallel  UseFilter=on  ControllerParametersSource=internal  P=1  I=1  D=0  N=100  b=1  c=1  InitialConditionSource=internal  InitialConditionForIntegrator=0  InitialConditionForFilter=0  ExternalReset=none  LimitOutput=off  UpperSaturationLimit=inf  LowerSaturationLimit=-inf  LinearizeAsGain=off  AntiWindupMode=none  Kb=1  TrackingMode=off  Kt=1  PParamMin=[]  PParamMax=[]  IParamMin=[]  IParamMax=[]  DParamMin=[]  DParamMax=[]  NParamMin=[]  NParamMax=[]  bParamMin=[]  bParamMax=[]  cParamMin=[]  cParamMax=[]  KbParamMin=[]  KbParamMax=[]  KtParamMin=[]  KtParamMax=[]  POutMin=[]  POutMax=[]  IOutMin=[]  IOutMax=[]  DOutMin=[]  DOutMax=[]  NOutMin=[]  NOutMax=[]  bOutMin=[]  bOutMax=[]  cOutMin=[]  cOutMax=[]  KbOutMin=[]  KbOutMax=[]  KtOutMin=[]  KtOutMax=[]  IntegratorOutMin=[]  IntegratorOutMax=[]  FilterOutMin=[]  FilterOutMax=[]  SumOutMin=[]  SumOutMax=[]  Sum1OutMin=[]  Sum1OutMax=[]  Sum2OutMin=[]  Sum2OutMax=[]  Sum3OutMin=[]  Sum3OutMax=[]  SumI1OutMin=[]  SumI1OutMax=[]  SumI2OutMin=[]  SumI2OutMax=[]  SumI3OutMin=[]  SumI3OutMax=[]  SumDOutMin=[]  SumDOutMax=[]  SaturationOutMin=[]  SaturationOutMax=[]  IntegratorContinuousStateAttributes=''  IntegratorStateMustResolveToSignalObject=off  IntegratorRTWStateStorageClass=Auto  FilterContinuousStateAttributes=''  FilterStateMustResolveToSignalObject=off  FilterRTWStateStorageClass=Auto  DifferentiatorICPrevScaledInput=0  DifferentiatorOutMin=[]  DifferentiatorOutMax=[]  InitialConditionSetting=State (most efficient)
  cfblk6 : simulink/Discrete/Transfer Fcn Real Zero  ZeroZ=0.75  ICPrevInput=0.0  DoSatur=off
      settings: SourceProductName=Simulink  SourceProductBaseCode=SL
  cfblk7 : simulink/Discrete/Transfer Fcn Lead or Lag  PoleZ=0.95  ZeroZ=0.75  ICPrevOutput=0.0  ICPrevInput=0.0  DoSatur=off
      settings: SourceProductName=Simulink  SourceProductBaseCode=SL
  cfblk8 : Delay  DelayLengthSource=Input port
      settings: InputPortMap=u0,p1
  cfblk9 : DiscreteFir
  cfblk2 : Outport
  wires:
  cfblk3/1 -> cfblk7/1
  cfblk5/1 -> cfblk6/1, cfblk22/1
  cfblk1/1 -> cfblk4/1
  cfblk4/1 -> cfblk13/1
  cfblk16/1 -> cfblk3/1
  cfblk8/1 -> cfblk11/1
  cfblk15/1 -> cfblk18/3(cfblk10)
  cfblk6/1 -> cfblk23/1, cfblk24/1
  cfblk10/1 -> cfblk2/1
  cfblk7/1 -> cfblk17/1(cfblk1)
  cfblk14/1 -> cfblk10/1
  cfblk12/1 -> cfblk9/1
  cfblk17/1(cfblk2) -> cfblk12/1
  cfblk17/2(cfblk17) -> cfblk8/2
  cfblk18/2(cfblk11) -> cfblk5/1
  cfblk13/1 -> cfblk17/Action
  cfblk13/2 -> cfblk18/Action
  cfblk9/1 -> cfblk19/1
  cfblk19/1 -> cfblk17/2(cfblk16)
  cfblk11/1 -> cfblk20/1
  cfblk20/1 -> cfblk18/2(cfblk9)
  cfblk18/1(cfblk2) -> cfblk21/1
  cfblk21/1 -> cfblk4/2
  cfblk22/1 -> cfblk18/1(cfblk1)
  cfblk23/1 -> cfblk8/1
  cfblk24/1 -> cfblk5/2

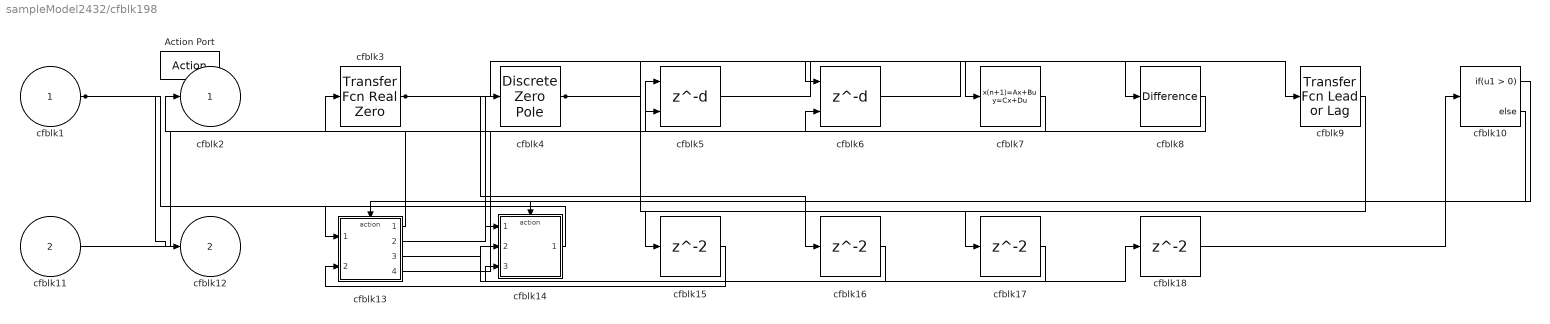
== system sampleModel2432/cfblk198 ==
  cfblk1 : Inport
  cfblk11 : Inport  Port=2
  Action Port : ActionPort  ActionType=else
  cfblk10 : If  SampleTime=1
  cfblk13 : Subsystem  TreatAsAtomicUnit=on
  cfblk14 : Subsystem  TreatAsAtomicUnit=on
  cfblk{15..18} (4 alike) : Delay
  cfblk3 : simulink/Discrete/Transfer Fcn Real Zero  ZeroZ=0.75  ICPrevInput=0.0  DoSatur=off
      settings: SourceProductName=Simulink  SourceProductBaseCode=SL
  cfblk4 : DiscreteZeroPole  Poles=[0 0.5]  Gain=1  SampleTime=-1
  cfblk5 : Delay  DelayLengthSource=Input port
      settings: InputPortMap=u0,p1
  cfblk6 : Delay  DelayLengthSource=Input port
      settings: InputPortMap=u0,p1
  cfblk7 : DiscreteStateSpace  SampleTime=-1
  cfblk8 : simulink/Discrete/Difference  ICPrevInput=0.0  OutMin=[]  OutMax=[]  OutDataTypeStr=Inherit: Inherit via back propagation  OutDataType=fixdt(1, 16)  OutScaling=2^-10  DoSatur=off
  cfblk9 : simulink/Discrete/Transfer Fcn Lead or Lag  PoleZ=0.95  ZeroZ=0.75  ICPrevOutput=0.0  ICPrevInput=0.0  DoSatur=off
      settings: SourceProductName=Simulink  SourceProductBaseCode=SL
  cfblk2 : Outport
  cfblk12 : Outport  Port=2
  wires:
  cfblk5/1 -> cfblk9/1
  cfblk8/1 -> cfblk5/1
  cfblk3/1 -> cfblk6/1, cfblk16/1
  cfblk14/1(cfblk2) -> cfblk13/1(cfblk1)
  cfblk7/1 -> cfblk2/1
  cfblk11/1 -> cfblk5/2
  cfblk1/1 -> cfblk12/1, cfblk14/1(cfblk1)
  cfblk4/1 -> cfblk7/1, cfblk17/1
  cfblk6/1 -> cfblk8/1
  cfblk13/1(cfblk2) -> cfblk3/1
  cfblk13/2(cfblk14) -> cfblk4/1
  cfblk13/4(cfblk16) -> cfblk6/2
  cfblk10/1 -> cfblk13/Action
  cfblk10/2 -> cfblk14/Action
  cfblk9/1 -> cfblk15/1
  cfblk15/1 -> cfblk13/2(cfblk13)
  cfblk16/1 -> cfblk14/3(cfblk12)
  cfblk17/1 -> cfblk14/2(cfblk11)
  cfblk13/3(cfblk15) -> cfblk18/1
  cfblk18/1 -> cfblk10/1

== system sampleModel2432/cfblk199 ==
  cfblk1 : Inport
  Action Port : ActionPort  ActionType=then
  cfblk10 : Delay  DelayLengthSource=Input port
      settings: InputPortMap=u0,p1
  cfblk3 : DiscreteFilter
  cfblk4 : DiscreteIntegrator  InitialConditionSetting=State (most efficient)  SampleTime=-1  ICPrevOutput=DiscIntNeverNeededParam  ICPrevScaledInput=DiscIntNeverNeededParam
  cfblk5 : Delay  ShowEnablePort=on
      settings: InputPortMap=u0,e6
  cfblk6 : simulink/Discrete/Transfer Fcn First Order  PoleZ=0.95  ICPrevOutput=0.0  DoSatur=off
      settings: SourceProductName=Simulink
  cfblk7 : simulink/Discrete/Tapped Delay  vinit=0.0  samptime=-1  NumDelays=1  DelayOrder=Oldest  includeCurrent=off
  cfblk8 : UnitDelay  SampleTime=-1
  cfblk9 : DiscreteZeroPole  Poles=[0 0.5]  Gain=1  SampleTime=-1
  cfblk2 : Outport
  cfblk11 : Outport  Port=2
  wires:
  cfblk5/1 -> cfblk3/1
  cfblk8/1 -> cfblk10/1
  cfblk10/1 -> cfblk9/1
  cfblk6/1 -> cfblk7/1, cfblk4/1
  cfblk7/1 -> cfblk8/1
  cfblk4/1 -> cfblk11/1, cfblk10/2, cfblk5/2
  cfblk3/1 -> cfblk2/1
  cfblk9/1 -> cfblk5/1
  cfblk1/1 -> cfblk6/1

== system sampleModel2432/cfblk200 ==
  cfblk1 : Inport
  cfblk8 : Inport  Port=2
  cfblk9 : Inport  Port=3
  Action Port : ActionPort  ActionType=else
  cfblk11 : Delay
  cfblk3 : UnitDelay  SampleTime=-1
  cfblk4 : DiscreteTransferFcn
  cfblk5 : DiscreteFilter
  cfblk6 : DiscreteFir
  cfblk7 : simulink/Discrete/Tapped Delay  vinit=0.0  samptime=-1  NumDelays=1  DelayOrder=Oldest  includeCurrent=off
  cfblk2 : Outport
  cfblk10 : Outport  Port=2
  wires:
  cfblk8/1 -> cfblk2/1
  cfblk6/1 -> cfblk4/1
  cfblk4/1 -> cfblk5/1
  cfblk3/1 -> cfblk7/1
  cfblk9/1 -> cfblk6/1
  cfblk5/1 -> cfblk10/1
  cfblk7/1 -> cfblk11/1
  cfblk11/1 -> cfblk3/1

== system sampleModel2432/cfblk201 ==
  cfblk1 : Inport
  cfblk11 : Inport  Port=2
  Action Port : ActionPort  ActionType=then
  cfblk{3,7..8,10} (4 alike) : DiscreteZeroPole  Poles=[0 0.5]  Gain=1  SampleTime=-1
  cfblk14 : Delay
  cfblk4 : simulink/Discrete/Difference  ICPrevInput=0.0  OutMin=[]  OutMax=[]  OutDataTypeStr=Inherit: Inherit via back propagation  OutDataType=fixdt(1, 16)  OutScaling=2^-10  DoSatur=off
  cfblk5 : simulink/Continuous/PID Controller  Controller=PID  TimeDomain=Discrete-time  SampleTime=-1  IntegratorMethod=Forward Euler  FilterMethod=Forward Euler  Form=Parallel  UseFilter=on  ControllerParametersSource=internal  P=1  I=1  D=0  N=100  InitialConditionSource=internal  InitialConditionForIntegrator=0  InitialConditionForFilter=0  ExternalReset=none  LimitOutput=off  UpperSaturationLimit=inf  LowerSaturationLimit=-inf  LinearizeAsGain=off  AntiWindupMode=none  Kb=1  TrackingMode=off  Kt=1  PParamMin=[]  PParamMax=[]  IParamMin=[]  IParamMax=[]  DParamMin=[]  DParamMax=[]  NParamMin=[]  NParamMax=[]  KbParamMin=[]  KbParamMax=[]  KtParamMin=[]  KtParamMax=[]  POutMin=[]  POutMax=[]  IOutMin=[]  IOutMax=[]  DOutMin=[]  DOutMax=[]  NOutMin=[]  NOutMax=[]  KbOutMin=[]  KbOutMax=[]  KtOutMin=[]  KtOutMax=[]  IntegratorOutMin=[]  IntegratorOutMax=[]  FilterOutMin=[]  FilterOutMax=[]  SumOutMin=[]  SumOutMax=[]  SumI1OutMin=[]  SumI1OutMax=[]  SumI2OutMin=[]  SumI2OutMax=[]  SumI3OutMin=[]  SumI3OutMax=[]  SumDOutMin=[]  SumDOutMax=[]  SaturationOutMin=[]  SaturationOutMax=[]  IntegratorContinuousStateAttributes=''  IntegratorStateMustResolveToSignalObject=off  IntegratorRTWStateStorageClass=Auto  FilterContinuousStateAttributes=''  FilterStateMustResolveToSignalObject=off  FilterRTWStateStorageClass=Auto  DifferentiatorICPrevScaledInput=0  DifferentiatorOutMin=[]  DifferentiatorOutMax=[]  InitialConditionSetting=State (most efficient)
  cfblk6 : Delay
  cfblk9 : DiscreteFir
  cfblk2 : Outport
  cfblk12 : Outport  Port=2
  cfblk13 : Outport  Port=3
  wires:
  cfblk1/1 -> cfblk2/1
  cfblk3/1 -> cfblk9/1
  cfblk5/1 -> cfblk6/1
  cfblk9/1 -> cfblk7/1
  cfblk10/1 -> cfblk13/1
  cfblk7/1 -> cfblk12/1
  cfblk8/1 -> cfblk3/1
  cfblk4/1 -> cfblk8/1, cfblk10/1
  cfblk11/1 -> cfblk4/1
  cfblk6/1 -> cfblk14/1
  cfblk14/1 -> cfblk5/1

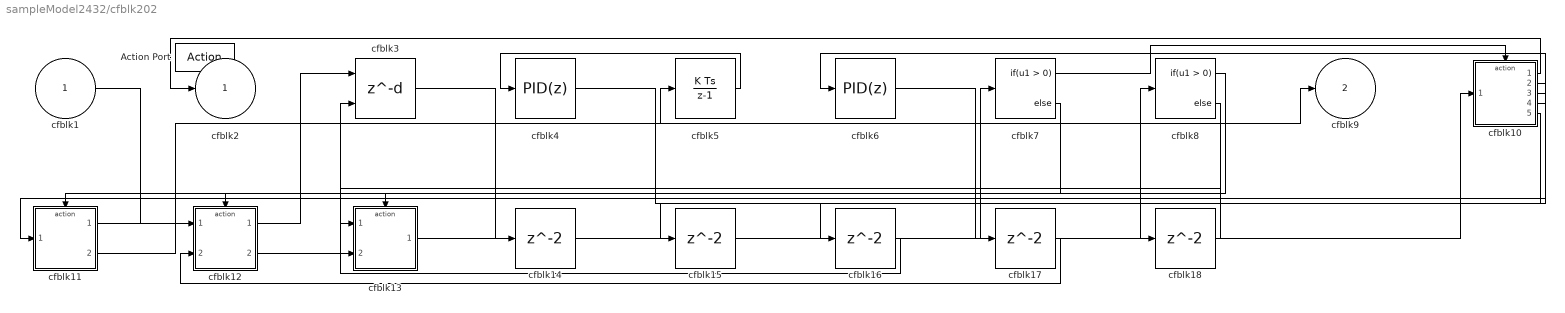
== system sampleModel2432/cfblk202 ==
  cfblk1 : Inport
  Action Port : ActionPort  ActionType=else
  cfblk10 : Subsystem  TreatAsAtomicUnit=on
  cfblk11 : Subsystem  TreatAsAtomicUnit=on
  cfblk12 : Subsystem  TreatAsAtomicUnit=on
  cfblk13 : Subsystem  TreatAsAtomicUnit=on
  cfblk{14..18} (5 alike) : Delay
  cfblk3 : Delay  DelayLengthSource=Input port
      settings: InputPortMap=u0,p1
  cfblk4 : simulink/Continuous/PID Controller  Controller=PID  TimeDomain=Discrete-time  SampleTime=-1  IntegratorMethod=Forward Euler  FilterMethod=Forward Euler  Form=Parallel  UseFilter=on  ControllerParametersSource=internal  P=1  I=1  D=0  N=100  InitialConditionSource=internal  InitialConditionForIntegrator=0  InitialConditionForFilter=0  ExternalReset=none  LimitOutput=off  UpperSaturationLimit=inf  LowerSaturationLimit=-inf  LinearizeAsGain=off  AntiWindupMode=none  Kb=1  TrackingMode=off  Kt=1  PParamMin=[]  PParamMax=[]  IParamMin=[]  IParamMax=[]  DParamMin=[]  DParamMax=[]  NParamMin=[]  NParamMax=[]  KbParamMin=[]  KbParamMax=[]  KtParamMin=[]  KtParamMax=[]  POutMin=[]  POutMax=[]  IOutMin=[]  IOutMax=[]  DOutMin=[]  DOutMax=[]  NOutMin=[]  NOutMax=[]  KbOutMin=[]  KbOutMax=[]  KtOutMin=[]  KtOutMax=[]  IntegratorOutMin=[]  IntegratorOutMax=[]  FilterOutMin=[]  FilterOutMax=[]  SumOutMin=[]  SumOutMax=[]  SumI1OutMin=[]  SumI1OutMax=[]  SumI2OutMin=[]  SumI2OutMax=[]  SumI3OutMin=[]  SumI3OutMax=[]  SumDOutMin=[]  SumDOutMax=[]  SaturationOutMin=[]  SaturationOutMax=[]  IntegratorContinuousStateAttributes=''  IntegratorStateMustResolveToSignalObject=off  IntegratorRTWStateStorageClass=Auto  FilterContinuousStateAttributes=''  FilterStateMustResolveToSignalObject=off  FilterRTWStateStorageClass=Auto  DifferentiatorICPrevScaledInput=0  DifferentiatorOutMin=[]  DifferentiatorOutMax=[]  InitialConditionSetting=State (most efficient)
  cfblk5 : DiscreteIntegrator  InitialConditionSetting=State (most efficient)  SampleTime=-1  ICPrevOutput=DiscIntNeverNeededParam  ICPrevScaledInput=DiscIntNeverNeededParam
  cfblk6 : simulink/Continuous/PID Controller  Controller=PID  TimeDomain=Discrete-time  SampleTime=-1  IntegratorMethod=Forward Euler  FilterMethod=Forward Euler  Form=Parallel  UseFilter=on  ControllerParametersSource=internal  P=1  I=1  D=0  N=100  InitialConditionSource=internal  InitialConditionForIntegrator=0  InitialConditionForFilter=0  ExternalReset=none  LimitOutput=off  UpperSaturationLimit=inf  LowerSaturationLimit=-inf  LinearizeAsGain=off  AntiWindupMode=none  Kb=1  TrackingMode=off  Kt=1  PParamMin=[]  PParamMax=[]  IParamMin=[]  IParamMax=[]  DParamMin=[]  DParamMax=[]  NParamMin=[]  NParamMax=[]  KbParamMin=[]  KbParamMax=[]  KtParamMin=[]  KtParamMax=[]  POutMin=[]  POutMax=[]  IOutMin=[]  IOutMax=[]  DOutMin=[]  DOutMax=[]  NOutMin=[]  NOutMax=[]  KbOutMin=[]  KbOutMax=[]  KtOutMin=[]  KtOutMax=[]  IntegratorOutMin=[]  IntegratorOutMax=[]  FilterOutMin=[]  FilterOutMax=[]  SumOutMin=[]  SumOutMax=[]  SumI1OutMin=[]  SumI1OutMax=[]  SumI2OutMin=[]  SumI2OutMax=[]  SumI3OutMin=[]  SumI3OutMax=[]  SumDOutMin=[]  SumDOutMax=[]  SaturationOutMin=[]  SaturationOutMax=[]  IntegratorContinuousStateAttributes=''  IntegratorStateMustResolveToSignalObject=off  IntegratorRTWStateStorageClass=Auto  FilterContinuousStateAttributes=''  FilterStateMustResolveToSignalObject=off  FilterRTWStateStorageClass=Auto  DifferentiatorICPrevScaledInput=0  DifferentiatorOutMin=[]  DifferentiatorOutMax=[]  InitialConditionSetting=State (most efficient)
  cfblk7 : If  SampleTime=1
  cfblk8 : If  SampleTime=1
  cfblk2 : Outport
  cfblk9 : Outport  Port=2
  wires:
  cfblk1/1 -> cfblk12/1(cfblk1)
  cfblk12/1(cfblk2) -> cfblk3/1
  cfblk12/2(cfblk16) -> cfblk3/2
  cfblk10/1(cfblk2) -> cfblk2/1
  cfblk10/3(cfblk10) -> cfblk6/1
  cfblk13/1(cfblk2) -> cfblk10/1(cfblk1)
  cfblk11/1(cfblk2) -> cfblk9/1
  cfblk5/1 -> cfblk4/1
  cfblk10/4(cfblk11) -> cfblk11/1(cfblk1)
  cfblk11/2(cfblk13) -> cfblk5/1
  cfblk7/1 -> cfblk10/Action
  cfblk7/2 -> cfblk11/Action
  cfblk8/1 -> cfblk12/Action
  cfblk8/2 -> cfblk13/Action
  cfblk3/1 -> cfblk14/1
  cfblk14/1 -> cfblk8/1
  cfblk10/2(cfblk9) -> cfblk15/1
  cfblk15/1 -> cfblk7/1
  cfblk4/1 -> cfblk16/1
  cfblk16/1 -> cfblk13/2(cfblk7)
  cfblk6/1 -> cfblk17/1
  cfblk17/1 -> cfblk12/2(cfblk15)
  cfblk10/5(cfblk12) -> cfblk18/1
  cfblk18/1 -> cfblk13/1(cfblk1)

== system sampleModel2432/cfblk203 ==
  cfblk1 : Inport
  cfblk13 : Inport  Port=2
  cfblk14 : Inport  Port=3
  Action Port : ActionPort  ActionType=then
  cfblk10 : simulink/Discrete/Difference  ICPrevInput=0.0  OutMin=[]  OutMax=[]  OutDataTypeStr=Inherit: Inherit via back propagation  OutDataType=fixdt(1, 16)  OutScaling=2^-10  DoSatur=off
  cfblk11 : DiscreteTransferFcn
  cfblk12 : simulink/Discrete/Tapped Delay  vinit=0.0  samptime=-1  NumDelays=1  DelayOrder=Oldest  includeCurrent=off
  cfblk3 : simulink/Continuous/PID Controller (2DOF)  Controller=PID  TimeDomain=Discrete-time  SampleTime=-1  IntegratorMethod=Forward Euler  FilterMethod=Forward Euler  Form=Parallel  UseFilter=on  ControllerParametersSource=internal  P=1  I=1  D=0  N=100  b=1  c=1  InitialConditionSource=internal  InitialConditionForIntegrator=0  InitialConditionForFilter=0  ExternalReset=none  LimitOutput=off  UpperSaturationLimit=inf  LowerSaturationLimit=-inf  LinearizeAsGain=off  AntiWindupMode=none  Kb=1  TrackingMode=off  Kt=1  PParamMin=[]  PParamMax=[]  IParamMin=[]  IParamMax=[]  DParamMin=[]  DParamMax=[]  NParamMin=[]  NParamMax=[]  bParamMin=[]  bParamMax=[]  cParamMin=[]  cParamMax=[]  KbParamMin=[]  KbParamMax=[]  KtParamMin=[]  KtParamMax=[]  POutMin=[]  POutMax=[]  IOutMin=[]  IOutMax=[]  DOutMin=[]  DOutMax=[]  NOutMin=[]  NOutMax=[]  bOutMin=[]  bOutMax=[]  cOutMin=[]  cOutMax=[]  KbOutMin=[]  KbOutMax=[]  KtOutMin=[]  KtOutMax=[]  IntegratorOutMin=[]  IntegratorOutMax=[]  FilterOutMin=[]  FilterOutMax=[]  SumOutMin=[]  SumOutMax=[]  Sum1OutMin=[]  Sum1OutMax=[]  Sum2OutMin=[]  Sum2OutMax=[]  Sum3OutMin=[]  Sum3OutMax=[]  SumI1OutMin=[]  SumI1OutMax=[]  SumI2OutMin=[]  SumI2OutMax=[]  SumI3OutMin=[]  SumI3OutMax=[]  SumDOutMin=[]  SumDOutMax=[]  SaturationOutMin=[]  SaturationOutMax=[]  IntegratorContinuousStateAttributes=''  IntegratorStateMustResolveToSignalObject=off  IntegratorRTWStateStorageClass=Auto  FilterContinuousStateAttributes=''  FilterStateMustResolveToSignalObject=off  FilterRTWStateStorageClass=Auto  DifferentiatorICPrevScaledInput=0  DifferentiatorOutMin=[]  DifferentiatorOutMax=[]  InitialConditionSetting=State (most efficient)
  cfblk4 : DiscreteZeroPole  Poles=[0 0.5]  Gain=1  SampleTime=-1
  cfblk5 : Delay  ShowEnablePort=on
      settings: InputPortMap=u0,e6
  cfblk6 : DiscreteIntegrator  InitialConditionSetting=State (most efficient)  SampleTime=-1  ICPrevOutput=DiscIntNeverNeededParam  ICPrevScaledInput=DiscIntNeverNeededParam
  cfblk7 : DiscreteFir
  cfblk8 : DiscreteZeroPole  Poles=[0 0.5]  Gain=1  SampleTime=-1
  cfblk9 : DiscreteZeroPole  Poles=[0 0.5]  Gain=1  SampleTime=-1
  cfblk2 : Outport
  cfblk15 : Outport  Port=2
  cfblk16 : Outport  Port=3
  wires:
  cfblk5/1 -> cfblk6/1
  cfblk12/1 -> cfblk15/1
  cfblk11/1 -> cfblk7/1
  cfblk4/1 -> cfblk10/1
  cfblk1/1 -> cfblk11/1
  cfblk9/1 -> cfblk4/1
  cfblk8/1 -> cfblk12/1
  cfblk3/1 -> cfblk2/1
  cfblk7/1 -> cfblk3/1, cfblk8/1
  cfblk10/1 -> cfblk5/1
  cfblk6/1 -> cfblk16/1
  cfblk14/1 -> cfblk3/2, cfblk9/1
  cfblk13/1 -> cfblk5/2

== system sampleModel2432/cfblk204 ==
  cfblk1 : Inport
  cfblk9 : Inport  Port=2
  cfblk10 : Inport  Port=3
  Action Port : ActionPort  ActionType=else
  cfblk13 : Subsystem  TreatAsAtomicUnit=on
  cfblk14 : Subsystem  TreatAsAtomicUnit=on
  cfblk15 : Delay
  cfblk16 : Delay
  cfblk3 : Delay
  cfblk4 : simulink/Discrete/Transfer Fcn Real Zero  ZeroZ=0.75  ICPrevInput=0.0  DoSatur=off
      settings: SourceProductName=Simulink  SourceProductBaseCode=SL
  cfblk5 : DiscreteFilter
  cfblk6 : DiscreteZeroPole  Poles=[0 0.5]  Gain=1  SampleTime=-1
  cfblk7 : DiscreteZeroPole  Poles=[0 0.5]  Gain=1  SampleTime=-1
  cfblk8 : If  SampleTime=1
  cfblk2 : Outport
  cfblk11 : Outport  Port=2
  cfblk12 : Outport  Port=3
  wires:
  cfblk5/1 -> cfblk3/1
  cfblk4/1 -> cfblk13/1(cfblk1)
  cfblk1/1 -> cfblk14/1(cfblk1)
  cfblk10/1 -> cfblk6/1
  cfblk14/1(cfblk2) -> cfblk5/1
  cfblk6/1 -> cfblk7/1
  cfblk7/1 -> cfblk4/1
  cfblk14/2(cfblk10) -> cfblk13/2(cfblk11)
  cfblk14/3(cfblk11) -> cfblk11/1
  cfblk14/4(cfblk12) -> cfblk12/1
  cfblk13/2(cfblk12) -> cfblk2/1
  cfblk8/1 -> cfblk13/Action
  cfblk8/2 -> cfblk14/Action
  cfblk3/1 -> cfblk15/1
  cfblk15/1 -> cfblk14/2(cfblk9)
  cfblk13/1(cfblk2) -> cfblk16/1
  cfblk16/1 -> cfblk8/1
